simulink library "JointHandler"  (R2016b)
settings: Solver=VariableStepAuto  StartTime=0.0  StopTime=10.0  RelTol=1e-3
undefined symbols (not defined in the file or in its folder): JointCommand, JointControlConfigLHFE, JointControlConfigLKFE, JointControlConfigRHFE, JointControlConfigRKFE, jointPolarityLHFE, jointPolarityLKFE, jointPolarityRHFE, jointPolarityRKFE, resolutionJointEncoder, zeroOffsetLHFE, zeroOffsetLKFE, zeroOffsetRHFE, zeroOffsetRKFE
libraries: simulink_extras x28, ConversionsLibrary x12, VariousLibrary x10, simulink x4, PositionSmoothener x1
settings Model: Creator=march  LastModifiedBy=march

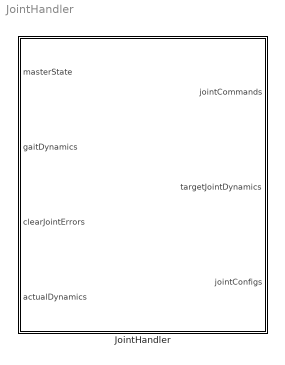
== system JointHandler ==
  JointHandler : Subsystem

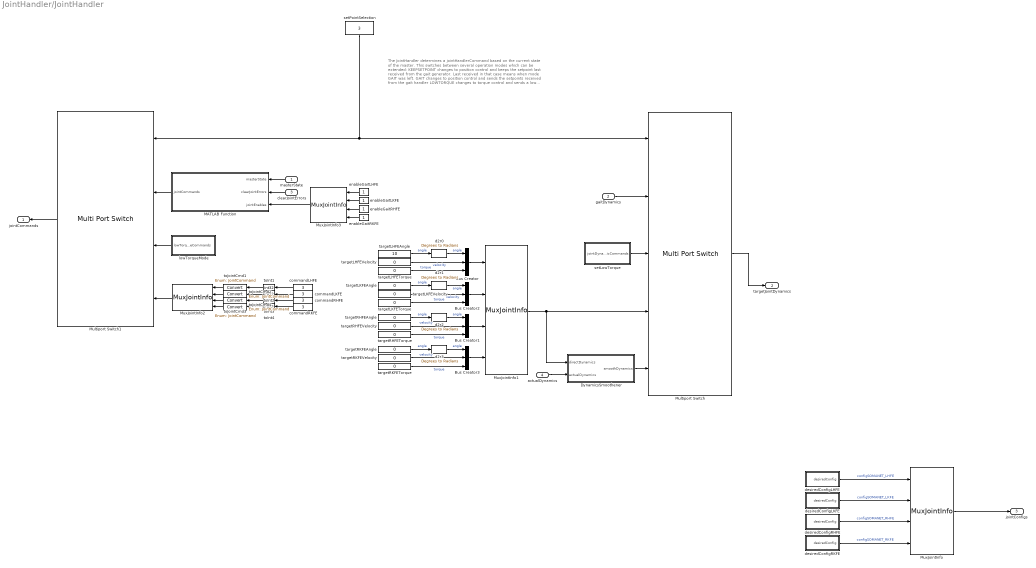
== system JointHandler/JointHandler ==
  note: The JointHandler determines a jointHandlerCommand based on the current
      | state of the master. This switches between several operation modes which
      | can be extended:
      | KEEPSETPOINT changes to position control and keeps the setpoint last
      | received from the gait generator. Last received in that case means when
      | mode GAIT was left.
      | GAIT changes to position control and sends the setpoints received from the
      | gait handler
      | LOWTORQUE changes to torque control and sends a low torque (50mNm)
      | to all joints
  masterState : Inport
  gaitDynamics : Inport  Port=2  OutDataTypeStr=Bus: JointDynamics
  clearJointErrors : Inport  Port=3
  actualDynamics : Inport  Port=4
  Bus Creator{,1..3} (4 alike) : BusCreator  Inputs=3  OutDataTypeStr=Bus: JointDynamics  NonVirtualBus=on
  DynamicsSmoothener : Subsystem
  MATLAB Function : MATLAB Function  TreatAsAtomicUnit=on
  Multiport Switch : MultiPortSwitch  DataPortOrder=Specify indices  DataPortIndices={1,2,3,4}  DiagnosticForDefault=Warning
  Multiport Switch1 : MultiPortSwitch  DataPortOrder=Specify indices  DataPortIndices={1,2,[3,4]}  DiagnosticForDefault=Warning
  MuxJointInfo{,1..3} (4 alike) : VariousLibrary/MuxJointInfo
  commandLHFE : Constant  Value=3
  commandLKFE : Constant  Value=3
  commandRHFE : Constant  Value=3
  commandRKFE : Constant  Value=3
  d2r{0..3} (4 alike) : simulink_extras/Transformations/Degrees to Radians
  desiredConfigLHFE : Subsystem
  desiredConfigLKFE : Subsystem
  desiredConfigRHFE : Subsystem
  desiredConfigRKFE : Subsystem
  enableGaitLHFE : Constant
  enableGaitLKFE : Constant
  enableGaitRHFE : Constant
  enableGaitRKFE : Constant
  lowTorqueMode : Subsystem
  setLowTorque : Subsystem
  setPointSelection : Constant  Value=3
  targetLHFEAngle : Constant  Value=10
  targetLHFETorque : Constant  Value=0
  targetLHFEVelocity : Constant  Value=0
  targetLKFEAngle : Constant  Value=0
  targetLKFETorque : Constant  Value=0
  targetLKFEVelocity : Constant  Value=0
  targetRHFEAngle : Constant  Value=0
  targetRHFETorque : Constant  Value=0
  targetRHFEVelocity : Constant  Value=0
  targetRKFEAngle : Constant  Value=0
  targetRKFETorque : Constant  Value=0
  targetRKFEVelocity : Constant  Value=0
  toInt{1..4} (4 alike) : DataTypeConversion  OutDataTypeStr=int32
  toJointCmd{1..4} (4 alike) : DataTypeConversion  OutDataTypeStr=Enum: JointCommand
  jointCommands : Outport
  "targetJointDynamics " : Outport  Port=2  OutDataTypeStr=Bus: JointDynamics  PortDimensions=[1 4]
  jointConfigs : Outport  Port=3  OutDataTypeStr=Bus: JointControlConfig  PortDimensions=[1 4]
  wires:
  MuxJointInfo3/1 -> MATLAB Function/3(jointEnables)
  enableGaitLHFE/1 -> MuxJointInfo3/1
  enableGaitLKFE/1 -> MuxJointInfo3/2
  enableGaitRKFE/1 -> MuxJointInfo3/4
  enableGaitRHFE/1 -> MuxJointInfo3/3
  commandRKFE/1 -> toInt4/1
  commandRHFE/1 -> toInt3/1
  commandLKFE/1 -> toInt2/1
  commandLHFE/1 -> toInt1/1
  toJointCmd4/1 -> MuxJointInfo2/4
  toJointCmd3/1 -> MuxJointInfo2/3
  toJointCmd2/1 -> MuxJointInfo2/2
  toInt4/1 -> toJointCmd4/1
  toInt3/1 -> toJointCmd3/1
  toInt2/1 -> toJointCmd2/1
  toJointCmd1/1 -> MuxJointInfo2/1
  toInt1/1 -> toJointCmd1/1
  Multiport Switch1/1 -> jointCommands/1
  Multiport Switch/1 -> "targetJointDynamics "/1
  MuxJointInfo2/1 -> Multiport Switch1/4
  lowTorqueMode/1(lowTorqueCommands) -> Multiport Switch1/3
  MATLAB Function/1(jointCommands) -> Multiport Switch1/2
  Bus Creator3/1 -> MuxJointInfo1/4
  Bus Creator1/1 -> MuxJointInfo1/3
  Bus Creator2/1 -> MuxJointInfo1/2
  Bus Creator/1 -> MuxJointInfo1/1
  d2r3/1 -> Bus Creator3/1  "angle"
  targetRKFEAngle/1 -> d2r3/1  "angle"
  targetRKFEVelocity/1 -> Bus Creator3/2  "velocity"
  targetRKFETorque/1 -> Bus Creator3/3  "torque"
  d2r2/1 -> Bus Creator1/1  "angle"
  targetRHFEAngle/1 -> d2r2/1  "angle"
  targetRHFEVelocity/1 -> Bus Creator1/2  "velocity"
  targetRHFETorque/1 -> Bus Creator1/3  "torque"
  MuxJointInfo1/1 -> Multiport Switch/4, DynamicsSmoothener/1(directDynamics)
  clearJointErrors/1 -> MATLAB Function/2(clearJointErrors)
  setLowTorque/1(jointDynamicCommands) -> Multiport Switch/3
  d2r1/1 -> Bus Creator2/1  "angle"
  d2r0/1 -> Bus Creator/1  "angle"
  desiredConfigLKFE/1(desiredConfig) -> MuxJointInfo/2  "configSOMANET_LKFE"
  desiredConfigLHFE/1(desiredConfig) -> MuxJointInfo/1  "configSOMANET_LHFE"
  desiredConfigRHFE/1(desiredConfig) -> MuxJointInfo/3  "configSOMANET_RHFE"
  desiredConfigRKFE/1(desiredConfig) -> MuxJointInfo/4  "configSOMANET_RKFE"
  MuxJointInfo/1 -> jointConfigs/1
  targetLKFEAngle/1 -> d2r1/1  "angle"
  targetLKFEVelocity/1 -> Bus Creator2/2  "velocity"
  targetLKFETorque/1 -> Bus Creator2/3  "torque"
  targetLHFEAngle/1 -> d2r0/1  "angle"
  targetLHFEVelocity/1 -> Bus Creator/2  "velocity"
  targetLHFETorque/1 -> Bus Creator/3  "torque"
  masterState/1 -> MATLAB Function/1(masterState)
  setPointSelection/1 -> Multiport Switch/1, Multiport Switch1/1
  actualDynamics/1 -> DynamicsSmoothener/2(actualDynamics)
  DynamicsSmoothener/1(smoothDynamics) -> Multiport Switch/5
  gaitDynamics/1 -> Multiport Switch/2

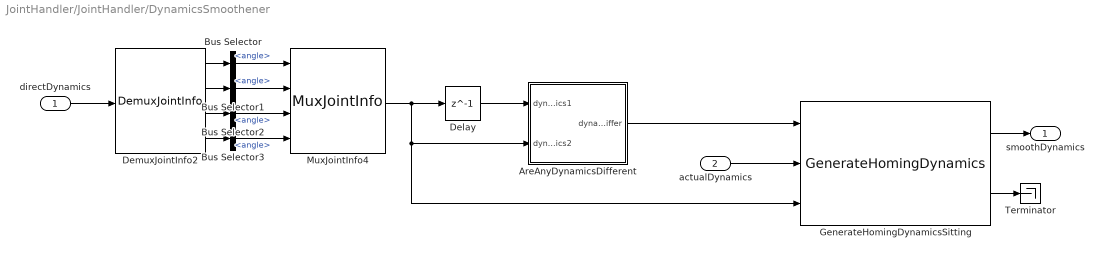
== system JointHandler/JointHandler/DynamicsSmoothener ==
  directDynamics : Inport
  actualDynamics : Inport  Port=2
  AreAnyDynamicsDifferent : Subsystem
  Bus Selector{,1..3} (4 alike) : BusSelector  OutputSignals=angle
  Delay : Delay  DelayLength=1
  DemuxJointInfo2 : VariousLibrary/DemuxJointInfo
  GenerateHomingDynamicsSitting : PositionSmoothener/GenerateHomingDynamics
  MuxJointInfo4 : VariousLibrary/MuxJointInfo
  Terminator : Terminator
  smoothDynamics : Outport
  wires:
  directDynamics/1 -> DemuxJointInfo2/1
  DemuxJointInfo2/1 -> Bus Selector/1
  DemuxJointInfo2/3 -> Bus Selector2/1
  DemuxJointInfo2/2 -> Bus Selector1/1
  DemuxJointInfo2/4 -> Bus Selector3/1
  GenerateHomingDynamicsSitting/2 -> Terminator/1
  GenerateHomingDynamicsSitting/1 -> smoothDynamics/1
  MuxJointInfo4/1 -> GenerateHomingDynamicsSitting/3, AreAnyDynamicsDifferent/2(dynamics2), Delay/1
  actualDynamics/1 -> GenerateHomingDynamicsSitting/2
  Bus Selector2/1 -> MuxJointInfo4/3  "<angle>"
  Bus Selector1/1 -> MuxJointInfo4/2  "<angle>"
  Bus Selector3/1 -> MuxJointInfo4/4  "<angle>"
  Bus Selector/1 -> MuxJointInfo4/1  "<angle>"
  Delay/1 -> AreAnyDynamicsDifferent/1(dynamics1)
  AreAnyDynamicsDifferent/1(dynamicsDiffer) -> GenerateHomingDynamicsSitting/1

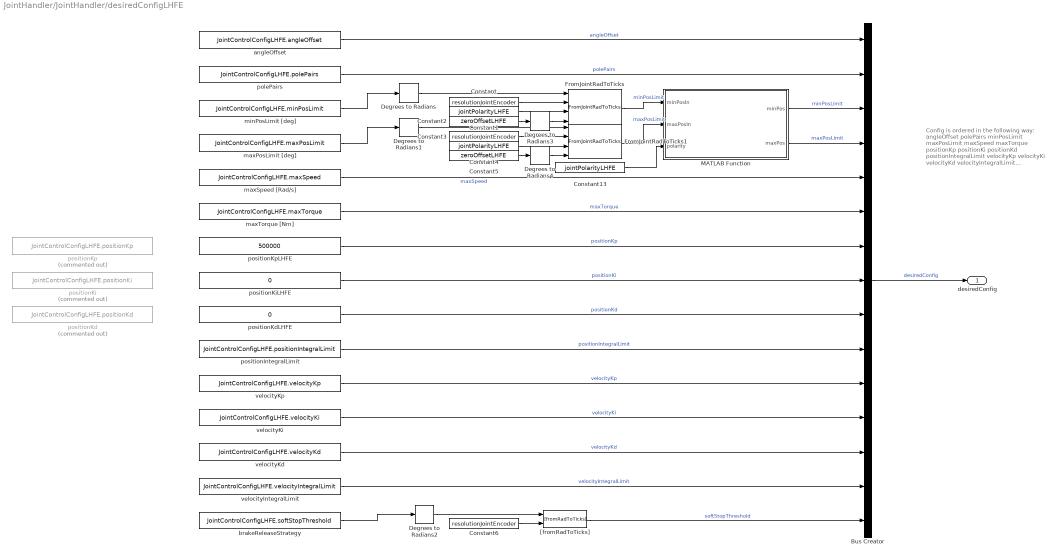
== system JointHandler/JointHandler/desiredConfigLHFE ==
  note: Config is ordered in the following way:
      | angleOffset
      | polePairs
      | minPosLimit
      | maxPosLimit
      | maxSpeed
      | maxTorque
      | positionKp
      | positionKi
      | positionKd
      | positionIntegralLimit
      | velocityKp
      | velocityKi
      | velocityKd
      | velocityIntegralLimit
      | brakeReleaseStrategy
  Bus Creator : BusCreator  Inputs=15  OutDataTypeStr=Bus: JointControlConfig  NonVirtualBus=on
  Constant : Constant  Value=resolutionJointEncoder
  Constant1 : Constant  Value=jointPolarityLHFE
  Constant13 : Constant  Value=jointPolarityLHFE
  Constant2 : Constant  Value=zeroOffsetLHFE
  Constant3 : Constant  Value=resolutionJointEncoder
  Constant4 : Constant  Value=jointPolarityLHFE
  Constant5 : Constant  Value=zeroOffsetLHFE
  Constant6 : Constant  Value=resolutionJointEncoder
  Degrees to Radians{,1..4} (5 alike) : simulink_extras/Transformations/Degrees to Radians
  FromJointRadToTicks : ConversionsLibrary/FromJointRadToTicks
  FromJointRadToTicks1 : ConversionsLibrary/FromJointRadToTicks
  MATLAB Function : MATLAB Function  TreatAsAtomicUnit=on
  "[fromRadToTicks]" : ConversionsLibrary/[fromRadToTicks]
  angleOffset : Constant  Value=JointControlConfigLHFE.angleOffset  OutDataTypeStr=double
  brakeReleaseStrategy : Constant  Value=JointControlConfigLHFE.softStopThreshold  OutDataTypeStr=double
  maxPosLimit [deg] : Constant  Value=JointControlConfigLHFE.maxPosLimit  OutDataTypeStr=double
  maxSpeed [Rad/s] : Constant  Value=JointControlConfigLHFE.maxSpeed  OutDataTypeStr=double
  maxTorque [Nm] : Constant  Value=JointControlConfigLHFE.maxTorque  OutDataTypeStr=double
  minPosLimit [deg] : Constant  Value=JointControlConfigLHFE.minPosLimit  OutDataTypeStr=double
  polePairs : Constant  Value=JointControlConfigLHFE.polePairs  OutMin=[0]  OutDataTypeStr=double
  positionIntegralLimit : Constant  Value=JointControlConfigLHFE.positionIntegralLimit  OutDataTypeStr=double
  positionKd : Constant  Commented=on  Value=JointControlConfigLHFE.positionKd  OutDataTypeStr=double
  positionKdLHFE : Constant  Value=0
  positionKi : Constant  Commented=on  Value=JointControlConfigLHFE.positionKi  OutDataTypeStr=double
  positionKiLHFE : Constant  Value=0
  positionKp : Constant  Commented=on  Value=JointControlConfigLHFE.positionKp  OutDataTypeStr=double
  positionKpLHFE : Constant  Value=500000
  velocityIntegralLimit : Constant  Value=JointControlConfigLHFE.velocityIntegralLimit  OutDataTypeStr=double
  velocityKd : Constant  Value=JointControlConfigLHFE.velocityKd  OutDataTypeStr=double
  velocityKi : Constant  Value=JointControlConfigLHFE.velocityKi  OutDataTypeStr=double
  velocityKp : Constant  Value=JointControlConfigLHFE.velocityKp  OutDataTypeStr=double
  desiredConfig : Outport  OutDataTypeStr=Bus: JointControlConfig
  wires:
  Constant13/1 -> MATLAB Function/3(polarity)
  FromJointRadToTicks1/1 -> MATLAB Function/2(maxPosIn)  "maxPosLimit"
  FromJointRadToTicks/1 -> MATLAB Function/1(minPosIn)  "minPosLimit"
  MATLAB Function/2(maxPos) -> Bus Creator/4  "maxPosLimit"
  MATLAB Function/1(minPos) -> Bus Creator/3  "minPosLimit"
  Degrees to Radians4/1 -> FromJointRadToTicks1/4
  Degrees to Radians3/1 -> FromJointRadToTicks/4
  brakeReleaseStrategy/1 -> Degrees to Radians2/1
  positionKdLHFE/1 -> Bus Creator/9  "positionKd"
  positionKiLHFE/1 -> Bus Creator/8  "positionKi"
  positionKpLHFE/1 -> Bus Creator/7  "positionKp"
  maxPosLimit [deg]/1 -> Degrees to Radians1/1
  minPosLimit [deg]/1 -> Degrees to Radians/1
  "[fromRadToTicks]"/1 -> Bus Creator/15  "softStopThreshold"
  Constant6/1 -> "[fromRadToTicks]"/2
  Degrees to Radians2/1 -> "[fromRadToTicks]"/1
  Constant3/1 -> FromJointRadToTicks1/2
  Constant4/1 -> FromJointRadToTicks1/3
  Constant5/1 -> Degrees to Radians4/1
  Constant/1 -> FromJointRadToTicks/2
  Constant1/1 -> FromJointRadToTicks/3
  Constant2/1 -> Degrees to Radians3/1
  Degrees to Radians1/1 -> FromJointRadToTicks1/1
  Degrees to Radians/1 -> FromJointRadToTicks/1
  maxSpeed [Rad/s]/1 -> Bus Creator/5  "maxSpeed"
  polePairs/1 -> Bus Creator/2  "polePairs"
  positionIntegralLimit/1 -> Bus Creator/10  "positionIntegralLimit"
  angleOffset/1 -> Bus Creator/1  "angleOffset"
  velocityIntegralLimit/1 -> Bus Creator/14  "velocityIntegralLimit"
  maxTorque [Nm]/1 -> Bus Creator/6  "maxTorque"
  velocityKp/1 -> Bus Creator/11  "velocityKp"
  velocityKi/1 -> Bus Creator/12  "velocityKi"
  velocityKd/1 -> Bus Creator/13  "velocityKd"
  Bus Creator/1 -> desiredConfig/1  "desiredConfig"

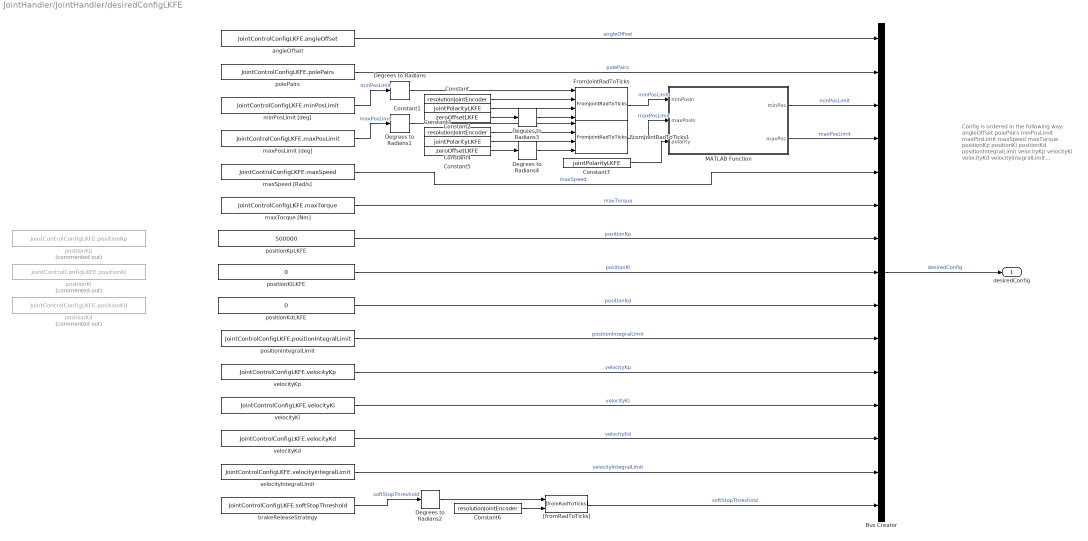
== system JointHandler/JointHandler/desiredConfigLKFE ==
  note: Config is ordered in the following way:
      | angleOffset
      | polePairs
      | minPosLimit
      | maxPosLimit
      | maxSpeed
      | maxTorque
      | positionKp
      | positionKi
      | positionKd
      | positionIntegralLimit
      | velocityKp
      | velocityKi
      | velocityKd
      | velocityIntegralLimit
      | brakeReleaseStrategy
  Bus Creator : BusCreator  Inputs=15  OutDataTypeStr=Bus: JointControlConfig  NonVirtualBus=on
  Constant : Constant  Value=resolutionJointEncoder
  Constant1 : Constant  Value=jointPolarityLKFE
  Constant2 : Constant  Value=zeroOffsetLKFE
  Constant3 : Constant  Value=resolutionJointEncoder
  Constant4 : Constant  Value=jointPolarityLKFE
  Constant5 : Constant  Value=zeroOffsetLKFE
  Constant6 : Constant  Value=resolutionJointEncoder
  Constant7 : Constant  Value=jointPolarityLKFE
  Degrees to Radians{,1..4} (5 alike) : simulink_extras/Transformations/Degrees to Radians
  FromJointRadToTicks : ConversionsLibrary/FromJointRadToTicks
  FromJointRadToTicks1 : ConversionsLibrary/FromJointRadToTicks
  MATLAB Function : MATLAB Function  TreatAsAtomicUnit=on
  "[fromRadToTicks]" : ConversionsLibrary/[fromRadToTicks]
  angleOffset : Constant  Value=JointControlConfigLKFE.angleOffset  OutDataTypeStr=double
  brakeReleaseStrategy : Constant  Value=JointControlConfigLKFE.softStopThreshold  OutDataTypeStr=double
  maxPosLimit [deg] : Constant  Value=JointControlConfigLKFE.maxPosLimit  OutDataTypeStr=double
  maxSpeed [Rad/s] : Constant  Value=JointControlConfigLKFE.maxSpeed  OutDataTypeStr=double
  maxTorque [Nm] : Constant  Value=JointControlConfigLKFE.maxTorque  OutDataTypeStr=double
  minPosLimit [deg] : Constant  Value=JointControlConfigLKFE.minPosLimit  OutDataTypeStr=double
  polePairs : Constant  Value=JointControlConfigLKFE.polePairs  OutMin=[0]  OutDataTypeStr=double
  positionIntegralLimit : Constant  Value=JointControlConfigLKFE.positionIntegralLimit  OutDataTypeStr=double
  positionKd : Constant  Commented=on  Value=JointControlConfigLKFE.positionKd  OutDataTypeStr=double
  positionKdLKFE : Constant  Value=0
  positionKi : Constant  Commented=on  Value=JointControlConfigLKFE.positionKi  OutDataTypeStr=double
  positionKiLKFE : Constant  Value=0
  positionKp : Constant  Commented=on  Value=JointControlConfigLKFE.positionKp  OutDataTypeStr=double
  positionKpLKFE : Constant  Value=500000
  velocityIntegralLimit : Constant  Value=JointControlConfigLKFE.velocityIntegralLimit  OutDataTypeStr=double
  velocityKd : Constant  Value=JointControlConfigLKFE.velocityKd  OutDataTypeStr=double
  velocityKi : Constant  Value=JointControlConfigLKFE.velocityKi  OutDataTypeStr=double
  velocityKp : Constant  Value=JointControlConfigLKFE.velocityKp  OutDataTypeStr=double
  desiredConfig : Outport  OutDataTypeStr=Bus: JointControlConfig
  wires:
  Constant7/1 -> MATLAB Function/3(polarity)
  FromJointRadToTicks1/1 -> MATLAB Function/2(maxPosIn)  "maxPosLimit"
  FromJointRadToTicks/1 -> MATLAB Function/1(minPosIn)  "minPosLimit"
  MATLAB Function/2(maxPos) -> Bus Creator/4  "maxPosLimit"
  MATLAB Function/1(minPos) -> Bus Creator/3  "minPosLimit"
  Degrees to Radians4/1 -> FromJointRadToTicks1/4
  Degrees to Radians3/1 -> FromJointRadToTicks/4
  brakeReleaseStrategy/1 -> Degrees to Radians2/1  "softStopThreshold"
  "[fromRadToTicks]"/1 -> Bus Creator/15  "softStopThreshold"
  Constant6/1 -> "[fromRadToTicks]"/2
  Degrees to Radians2/1 -> "[fromRadToTicks]"/1
  Constant3/1 -> FromJointRadToTicks1/2
  Constant4/1 -> FromJointRadToTicks1/3
  Constant5/1 -> Degrees to Radians4/1
  Constant/1 -> FromJointRadToTicks/2
  Constant1/1 -> FromJointRadToTicks/3
  Constant2/1 -> Degrees to Radians3/1
  Degrees to Radians1/1 -> FromJointRadToTicks1/1
  Degrees to Radians/1 -> FromJointRadToTicks/1
  Bus Creator/1 -> desiredConfig/1  "desiredConfig"
  angleOffset/1 -> Bus Creator/1  "angleOffset"
  polePairs/1 -> Bus Creator/2  "polePairs"
  minPosLimit [deg]/1 -> Degrees to Radians/1  "minPosLimit"
  maxPosLimit [deg]/1 -> Degrees to Radians1/1  "maxPosLimit"
  maxSpeed [Rad/s]/1 -> Bus Creator/5  "maxSpeed"
  maxTorque [Nm]/1 -> Bus Creator/6  "maxTorque"
  positionKpLKFE/1 -> Bus Creator/7  "positionKp"
  positionKiLKFE/1 -> Bus Creator/8  "positionKi"
  positionKdLKFE/1 -> Bus Creator/9  "positionKd"
  positionIntegralLimit/1 -> Bus Creator/10  "positionIntegralLimit"
  velocityKp/1 -> Bus Creator/11  "velocityKp"
  velocityKi/1 -> Bus Creator/12  "velocityKi"
  velocityKd/1 -> Bus Creator/13  "velocityKd"
  velocityIntegralLimit/1 -> Bus Creator/14  "velocityIntegralLimit"

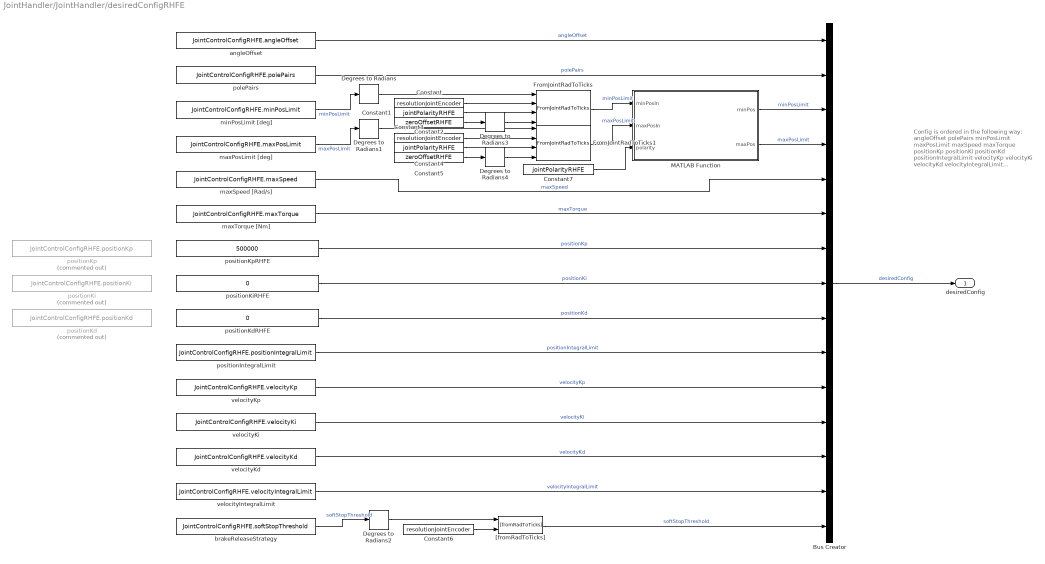
== system JointHandler/JointHandler/desiredConfigRHFE ==
  note: Config is ordered in the following way:
      | angleOffset
      | polePairs
      | minPosLimit
      | maxPosLimit
      | maxSpeed
      | maxTorque
      | positionKp
      | positionKi
      | positionKd
      | positionIntegralLimit
      | velocityKp
      | velocityKi
      | velocityKd
      | velocityIntegralLimit
      | brakeReleaseStrategy
  Bus Creator : BusCreator  Inputs=15  OutDataTypeStr=Bus: JointControlConfig  NonVirtualBus=on
  Constant : Constant  Value=resolutionJointEncoder
  Constant1 : Constant  Value=jointPolarityRHFE
  Constant2 : Constant  Value=zeroOffsetRHFE
  Constant3 : Constant  Value=resolutionJointEncoder
  Constant4 : Constant  Value=jointPolarityRHFE
  Constant5 : Constant  Value=zeroOffsetRHFE
  Constant6 : Constant  Value=resolutionJointEncoder
  Constant7 : Constant  Value=jointPolarityRHFE
  Degrees to Radians{,1..4} (5 alike) : simulink_extras/Transformations/Degrees to Radians
  FromJointRadToTicks : ConversionsLibrary/FromJointRadToTicks
  FromJointRadToTicks1 : ConversionsLibrary/FromJointRadToTicks
  MATLAB Function : MATLAB Function  TreatAsAtomicUnit=on
  "[fromRadToTicks]" : ConversionsLibrary/[fromRadToTicks]
  angleOffset : Constant  Value=JointControlConfigRHFE.angleOffset  OutDataTypeStr=double
  brakeReleaseStrategy : Constant  Value=JointControlConfigRHFE.softStopThreshold  OutDataTypeStr=double
  maxPosLimit [deg] : Constant  Value=JointControlConfigRHFE.maxPosLimit  OutDataTypeStr=double
  maxSpeed [Rad/s] : Constant  Value=JointControlConfigRHFE.maxSpeed  OutDataTypeStr=double
  maxTorque [Nm] : Constant  Value=JointControlConfigRHFE.maxTorque  OutDataTypeStr=double
  minPosLimit [deg] : Constant  Value=JointControlConfigRHFE.minPosLimit  OutDataTypeStr=double
  polePairs : Constant  Value=JointControlConfigRHFE.polePairs  OutMin=[0]  OutDataTypeStr=double
  positionIntegralLimit : Constant  Value=JointControlConfigRHFE.positionIntegralLimit  OutDataTypeStr=double
  positionKd : Constant  Commented=on  Value=JointControlConfigRHFE.positionKd  OutDataTypeStr=double
  positionKdRHFE : Constant  Value=0
  positionKi : Constant  Commented=on  Value=JointControlConfigRHFE.positionKi  OutDataTypeStr=double
  positionKiRHFE : Constant  Value=0
  positionKp : Constant  Commented=on  Value=JointControlConfigRHFE.positionKp  OutDataTypeStr=double
  positionKpRHFE : Constant  Value=500000
  velocityIntegralLimit : Constant  Value=JointControlConfigRHFE.velocityIntegralLimit  OutDataTypeStr=double
  velocityKd : Constant  Value=JointControlConfigRHFE.velocityKd  OutDataTypeStr=double
  velocityKi : Constant  Value=JointControlConfigRHFE.velocityKi  OutDataTypeStr=double
  velocityKp : Constant  Value=JointControlConfigRHFE.velocityKp  OutDataTypeStr=double
  desiredConfig : Outport  OutDataTypeStr=Bus: JointControlConfig
  wires:
  Constant7/1 -> MATLAB Function/3(polarity)
  FromJointRadToTicks1/1 -> MATLAB Function/2(maxPosIn)  "maxPosLimit"
  FromJointRadToTicks/1 -> MATLAB Function/1(minPosIn)  "minPosLimit"
  MATLAB Function/2(maxPos) -> Bus Creator/4  "maxPosLimit"
  MATLAB Function/1(minPos) -> Bus Creator/3  "minPosLimit"
  Degrees to Radians4/1 -> FromJointRadToTicks1/4
  Degrees to Radians3/1 -> FromJointRadToTicks/4
  brakeReleaseStrategy/1 -> Degrees to Radians2/1  "softStopThreshold"
  "[fromRadToTicks]"/1 -> Bus Creator/15  "softStopThreshold"
  Constant6/1 -> "[fromRadToTicks]"/2
  Degrees to Radians2/1 -> "[fromRadToTicks]"/1
  Constant3/1 -> FromJointRadToTicks1/2
  Constant4/1 -> FromJointRadToTicks1/3
  Constant5/1 -> Degrees to Radians4/1
  Constant/1 -> FromJointRadToTicks/2
  Constant1/1 -> FromJointRadToTicks/3
  Constant2/1 -> Degrees to Radians3/1
  Degrees to Radians1/1 -> FromJointRadToTicks1/1
  Degrees to Radians/1 -> FromJointRadToTicks/1
  Bus Creator/1 -> desiredConfig/1  "desiredConfig"
  angleOffset/1 -> Bus Creator/1  "angleOffset"
  polePairs/1 -> Bus Creator/2  "polePairs"
  minPosLimit [deg]/1 -> Degrees to Radians/1  "minPosLimit"
  maxPosLimit [deg]/1 -> Degrees to Radians1/1  "maxPosLimit"
  maxSpeed [Rad/s]/1 -> Bus Creator/5  "maxSpeed"
  maxTorque [Nm]/1 -> Bus Creator/6  "maxTorque"
  positionKpRHFE/1 -> Bus Creator/7  "positionKp"
  positionKiRHFE/1 -> Bus Creator/8  "positionKi"
  positionKdRHFE/1 -> Bus Creator/9  "positionKd"
  positionIntegralLimit/1 -> Bus Creator/10  "positionIntegralLimit"
  velocityKp/1 -> Bus Creator/11  "velocityKp"
  velocityKi/1 -> Bus Creator/12  "velocityKi"
  velocityKd/1 -> Bus Creator/13  "velocityKd"
  velocityIntegralLimit/1 -> Bus Creator/14  "velocityIntegralLimit"

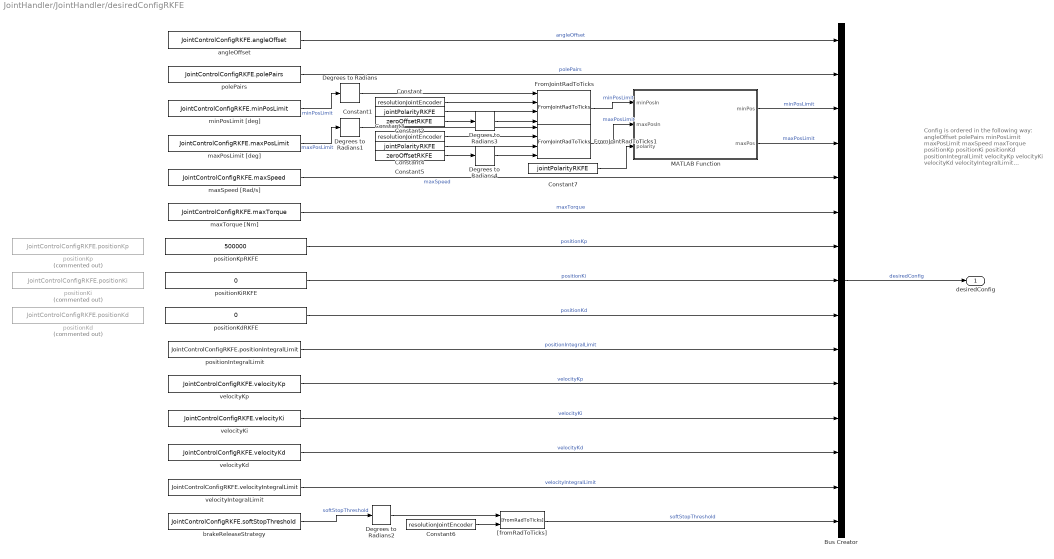
== system JointHandler/JointHandler/desiredConfigRKFE ==
  note: Config is ordered in the following way:
      | angleOffset
      | polePairs
      | minPosLimit
      | maxPosLimit
      | maxSpeed
      | maxTorque
      | positionKp
      | positionKi
      | positionKd
      | positionIntegralLimit
      | velocityKp
      | velocityKi
      | velocityKd
      | velocityIntegralLimit
      | brakeReleaseStrategy
  Bus Creator : BusCreator  Inputs=15  OutDataTypeStr=Bus: JointControlConfig  NonVirtualBus=on
  Constant : Constant  Value=resolutionJointEncoder
  Constant1 : Constant  Value=jointPolarityRKFE
  Constant2 : Constant  Value=zeroOffsetRKFE
  Constant3 : Constant  Value=resolutionJointEncoder
  Constant4 : Constant  Value=jointPolarityRKFE
  Constant5 : Constant  Value=zeroOffsetRKFE
  Constant6 : Constant  Value=resolutionJointEncoder
  Constant7 : Constant  Value=jointPolarityRKFE
  Degrees to Radians{,1..4} (5 alike) : simulink_extras/Transformations/Degrees to Radians
  FromJointRadToTicks : ConversionsLibrary/FromJointRadToTicks
  FromJointRadToTicks1 : ConversionsLibrary/FromJointRadToTicks
  MATLAB Function : MATLAB Function  TreatAsAtomicUnit=on
  "[fromRadToTicks]" : ConversionsLibrary/[fromRadToTicks]
  angleOffset : Constant  Value=JointControlConfigRKFE.angleOffset  OutDataTypeStr=double
  brakeReleaseStrategy : Constant  Value=JointControlConfigRKFE.softStopThreshold  OutDataTypeStr=double
  maxPosLimit [deg] : Constant  Value=JointControlConfigRKFE.maxPosLimit  OutDataTypeStr=double
  maxSpeed [Rad/s] : Constant  Value=JointControlConfigRKFE.maxSpeed  OutDataTypeStr=double
  maxTorque [Nm] : Constant  Value=JointControlConfigRKFE.maxTorque  OutDataTypeStr=double
  minPosLimit [deg] : Constant  Value=JointControlConfigRKFE.minPosLimit  OutDataTypeStr=double
  polePairs : Constant  Value=JointControlConfigRKFE.polePairs  OutMin=[0]  OutDataTypeStr=double
  positionIntegralLimit : Constant  Value=JointControlConfigRKFE.positionIntegralLimit  OutDataTypeStr=double
  positionKd : Constant  Commented=on  Value=JointControlConfigRKFE.positionKd  OutDataTypeStr=double
  positionKdRKFE : Constant  Value=0
  positionKi : Constant  Commented=on  Value=JointControlConfigRKFE.positionKi  OutDataTypeStr=double
  positionKiRKFE : Constant  Value=0
  positionKp : Constant  Commented=on  Value=JointControlConfigRKFE.positionKp  OutDataTypeStr=double
  positionKpRKFE : Constant  Value=500000
  velocityIntegralLimit : Constant  Value=JointControlConfigRKFE.velocityIntegralLimit  OutDataTypeStr=double
  velocityKd : Constant  Value=JointControlConfigRKFE.velocityKd  OutDataTypeStr=double
  velocityKi : Constant  Value=JointControlConfigRKFE.velocityKi  OutDataTypeStr=double
  velocityKp : Constant  Value=JointControlConfigRKFE.velocityKp  OutDataTypeStr=double
  desiredConfig : Outport  OutDataTypeStr=Bus: JointControlConfig
  wires:
  Constant7/1 -> MATLAB Function/3(polarity)
  FromJointRadToTicks1/1 -> MATLAB Function/2(maxPosIn)  "maxPosLimit"
  FromJointRadToTicks/1 -> MATLAB Function/1(minPosIn)  "minPosLimit"
  MATLAB Function/2(maxPos) -> Bus Creator/4  "maxPosLimit"
  MATLAB Function/1(minPos) -> Bus Creator/3  "minPosLimit"
  Degrees to Radians4/1 -> FromJointRadToTicks1/4
  Degrees to Radians3/1 -> FromJointRadToTicks/4
  brakeReleaseStrategy/1 -> Degrees to Radians2/1  "softStopThreshold"
  "[fromRadToTicks]"/1 -> Bus Creator/15  "softStopThreshold"
  Constant6/1 -> "[fromRadToTicks]"/2
  Degrees to Radians2/1 -> "[fromRadToTicks]"/1
  Constant3/1 -> FromJointRadToTicks1/2
  Constant4/1 -> FromJointRadToTicks1/3
  Constant5/1 -> Degrees to Radians4/1
  Constant/1 -> FromJointRadToTicks/2
  Constant1/1 -> FromJointRadToTicks/3
  Constant2/1 -> Degrees to Radians3/1
  Degrees to Radians1/1 -> FromJointRadToTicks1/1
  Degrees to Radians/1 -> FromJointRadToTicks/1
  Bus Creator/1 -> desiredConfig/1  "desiredConfig"
  angleOffset/1 -> Bus Creator/1  "angleOffset"
  polePairs/1 -> Bus Creator/2  "polePairs"
  minPosLimit [deg]/1 -> Degrees to Radians/1  "minPosLimit"
  maxPosLimit [deg]/1 -> Degrees to Radians1/1  "maxPosLimit"
  maxSpeed [Rad/s]/1 -> Bus Creator/5  "maxSpeed"
  maxTorque [Nm]/1 -> Bus Creator/6  "maxTorque"
  positionKpRKFE/1 -> Bus Creator/7  "positionKp"
  positionKiRKFE/1 -> Bus Creator/8  "positionKi"
  positionKdRKFE/1 -> Bus Creator/9  "positionKd"
  positionIntegralLimit/1 -> Bus Creator/10  "positionIntegralLimit"
  velocityKp/1 -> Bus Creator/11  "velocityKp"
  velocityKi/1 -> Bus Creator/12  "velocityKi"
  velocityKd/1 -> Bus Creator/13  "velocityKd"
  velocityIntegralLimit/1 -> Bus Creator/14  "velocityIntegralLimit"

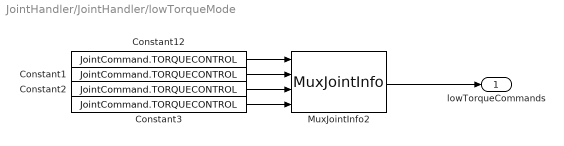
== system JointHandler/JointHandler/lowTorqueMode ==
  Constant{1..3,12} (4 alike) : Constant  Value=JointCommand.TORQUECONTROL
  MuxJointInfo2 : VariousLibrary/MuxJointInfo
  lowTorqueCommands : Outport
  wires:
  MuxJointInfo2/1 -> lowTorqueCommands/1
  Constant2/1 -> MuxJointInfo2/3
  Constant3/1 -> MuxJointInfo2/4
  Constant1/1 -> MuxJointInfo2/2
  Constant12/1 -> MuxJointInfo2/1

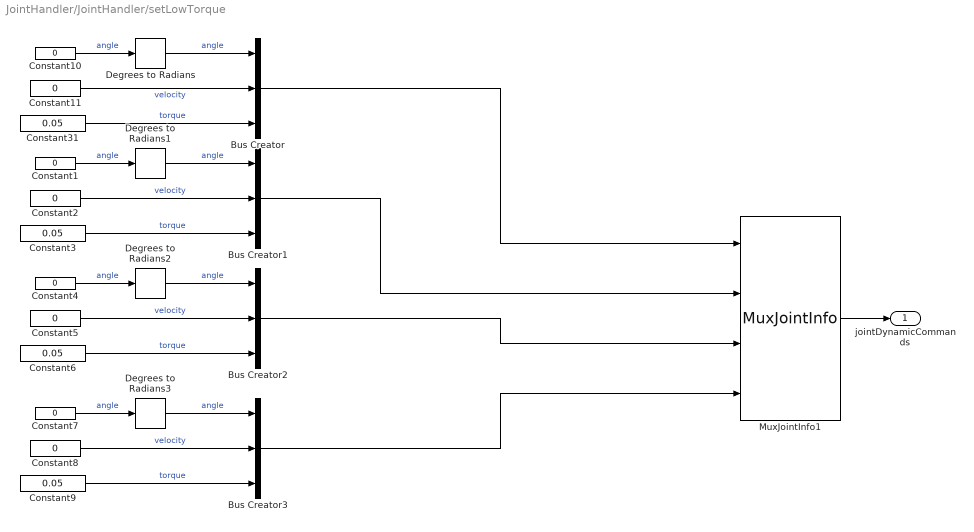
== system JointHandler/JointHandler/setLowTorque ==
  Bus Creator{,1..3} (4 alike) : BusCreator  Inputs=3  OutDataTypeStr=Bus: JointDynamics  NonVirtualBus=on
  Constant{1..2,4..5,7..8,10..11} (8 alike) : Constant  Value=0
  Constant{3,6,9,31} (4 alike) : Constant  Value=0.05
  Degrees to Radians{,1..3} (4 alike) : simulink_extras/Transformations/Degrees to Radians
  MuxJointInfo1 : VariousLibrary/MuxJointInfo
  jointDynamicCommands : Outport  OutDataTypeStr=Bus: JointDynamics  PortDimensions=[1 4]
  wires:
  Bus Creator3/1 -> MuxJointInfo1/4
  Bus Creator2/1 -> MuxJointInfo1/3
  Bus Creator1/1 -> MuxJointInfo1/2
  Bus Creator/1 -> MuxJointInfo1/1
  Constant9/1 -> Bus Creator3/3  "torque"
  Degrees to Radians3/1 -> Bus Creator3/1  "angle"
  Constant7/1 -> Degrees to Radians3/1  "angle"
  Constant8/1 -> Bus Creator3/2  "velocity"
  Constant6/1 -> Bus Creator2/3  "torque"
  Degrees to Radians2/1 -> Bus Creator2/1  "angle"
  Constant4/1 -> Degrees to Radians2/1  "angle"
  Constant5/1 -> Bus Creator2/2  "velocity"
  Constant3/1 -> Bus Creator1/3  "torque"
  Degrees to Radians1/1 -> Bus Creator1/1  "angle"
  Constant1/1 -> Degrees to Radians1/1  "angle"
  Constant2/1 -> Bus Creator1/2  "velocity"
  Constant31/1 -> Bus Creator/3  "torque"
  Degrees to Radians/1 -> Bus Creator/1  "angle"
  Constant10/1 -> Degrees to Radians/1  "angle"
  Constant11/1 -> Bus Creator/2  "velocity"
  MuxJointInfo1/1 -> jointDynamicCommands/1

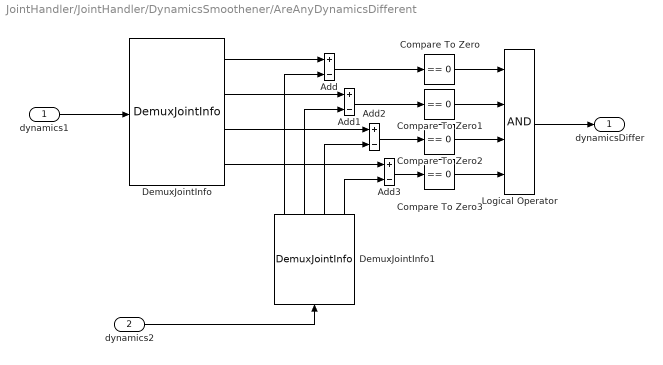
== system JointHandler/JointHandler/DynamicsSmoothener/AreAnyDynamicsDifferent ==
  dynamics1 : Inport
  dynamics2 : Inport  Port=2
  Add{,1..3} (4 alike) : Sum  Inputs=+-
  Compare To Zero{,1..3} (4 alike) : simulink/Logic and Bit Operations/Compare To Zero  relop===  OutDataTypeStr=boolean
  DemuxJointInfo : VariousLibrary/DemuxJointInfo
  DemuxJointInfo1 : VariousLibrary/DemuxJointInfo
  Logical Operator : Logic  Inputs=4  AllPortsSameDT=off  OutDataTypeStr=boolean
  dynamicsDiffer : Outport
  wires:
  dynamics2/1 -> DemuxJointInfo1/1
  DemuxJointInfo1/4 -> Add3/2
  dynamics1/1 -> DemuxJointInfo/1
  Add3/1 -> Compare To Zero3/1
  DemuxJointInfo1/1 -> Add/2
  Compare To Zero/1 -> Logical Operator/1
  Compare To Zero1/1 -> Logical Operator/2
  Compare To Zero2/1 -> Logical Operator/3
  Logical Operator/1 -> dynamicsDiffer/1
  Add2/1 -> Compare To Zero2/1
  DemuxJointInfo1/3 -> Add2/2
  DemuxJointInfo/4 -> Add3/1
  DemuxJointInfo/3 -> Add2/1
  Compare To Zero3/1 -> Logical Operator/4
  DemuxJointInfo1/2 -> Add1/2
  DemuxJointInfo/2 -> Add1/1
  Add1/1 -> Compare To Zero1/1
  Add/1 -> Compare To Zero/1
  DemuxJointInfo/1 -> Add/1

== matlab function JointHandler/MATLAB Function ==
  data: masterState input; jointCommands output; clearJointErrors input; jointEnables input
function jointCommands   = getJointCommandsFromState( masterState, clearJointErrors, jointEnables )
% wrapper for getJointCommandsFromState
[ jointCommands ] = getJointCommandsFromState( masterState, clearJointErrors, jointEnables );
end

== matlab function JointHandler/desiredConfigRKFE/MATLAB Function ==
  data: minPosIn input; minPos output; maxPosIn input; polarity input; maxPos output
function [ minPos, maxPos ] = getMinMaxWithPolarity( minPosIn, maxPosIn, polarity )
%wrapper for getMinMaxWithPolarity
[ minPos, maxPos ] = getMinMaxWithPolarity( minPosIn, maxPosIn, polarity );
end

== matlab function JointHandler/desiredConfigRHFE/MATLAB Function ==
  data: minPosIn input; minPos output; maxPosIn input; polarity input; maxPos output
function [ minPos, maxPos ] = getMinMaxWithPolarity( minPosIn, maxPosIn, polarity )
%wrapper for getMinMaxWithPolarity
[ minPos, maxPos ] = getMinMaxWithPolarity( minPosIn, maxPosIn, polarity );
end

== matlab function JointHandler/desiredConfigLKFE/MATLAB Function ==
  data: minPosIn input; minPos output; maxPosIn input; polarity input; maxPos output
function [ minPos, maxPos ] = getMinMaxWithPolarity( minPosIn, maxPosIn, polarity )
%wrapper for getMinMaxWithPolarity
[ minPos, maxPos ] = getMinMaxWithPolarity( minPosIn, maxPosIn, polarity );
end

== matlab function JointHandler/desiredConfigLHFE/MATLAB Function ==
  data: minPosIn input; minPos output; maxPosIn input; polarity input; maxPos output
function [ minPos, maxPos ] = getMinMaxWithPolarity( minPosIn, maxPosIn, polarity )
%wrapper for getMinMaxWithPolarity
[ minPos, maxPos ] = getMinMaxWithPolarity( minPosIn, maxPosIn, polarity );
end
